simulink model "inner_pid_discrete_test"  (R2016a)
settings: Solver=VariableStepAuto  StartTime=0.0  StopTime=50  RelTol=1e-3
values from neighbouring files (symbols this model uses):
  max_ang_ref = 0.5    [init.m]
  PosD = 0.24    [init.m]
  PosI = 0    [init.m]
  PosP = 0.20    (= 0.2)    [init.m]
undefined symbols (not defined in the file or in its folder): b, inner_h, inner_maxlim, inner_minlim, k, l
libraries: simulink x7, vrlib x2

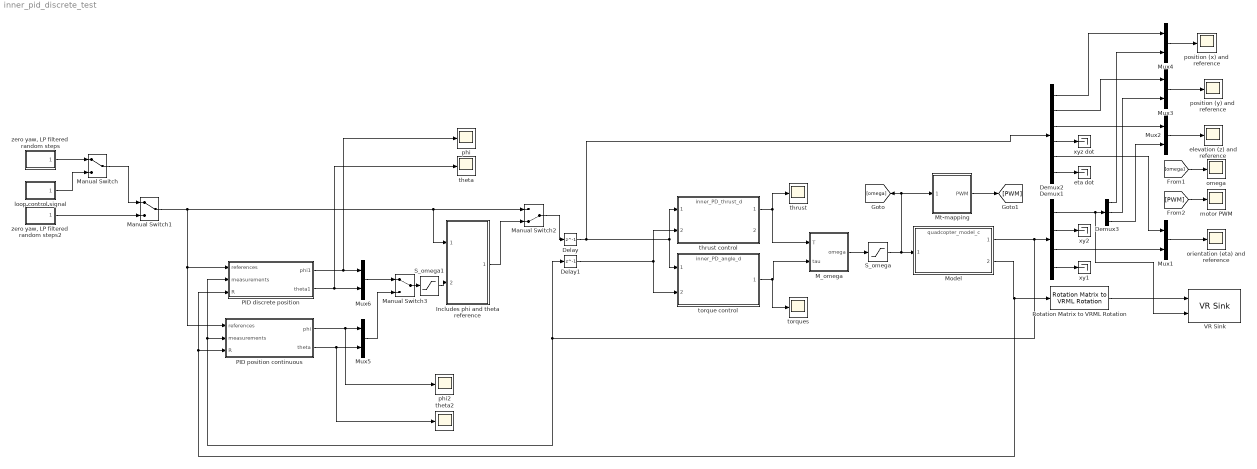
== system inner_pid_discrete_test ==
  "   eta dot" : Terminator
  "   xy1" : Terminator
  "   xy2" : Terminator
  "  xyz dot" : Terminator
  Delay : Delay  DelayLength=1  InitialCondition=0  SampleTime=inner_h
  Delay1 : Delay  DelayLength=1  InitialCondition=0  SampleTime=inner_h
  Demux1 : Demux  Outputs=[3,3,3,3]
  Demux2 : Demux  Outputs=[1,1,1,3,3,3]
  Demux3 : Demux  Outputs=[1,1,1]
  Includes phi and theta reference : Subsystem
  M_omega : Subsystem
  Manual Switch : ManualSwitch
  Manual Switch1 : ManualSwitch
  Manual Switch2 : ManualSwitch  CurrentSetting=0
  Manual Switch3 : ManualSwitch
  Model : ModelReference  ModelNameDialog=quadcopter_model_c.mdl  SimulationMode=Normal  ModelReferenceVersion=1.156
  Mt-mapping : Subsystem
  Mux{1..6} (6 alike) : Mux  Inputs=2
  PID discrete position : Subsystem
  PID position continuous : Subsystem
  Rotation Matrix to VRML Rotation : vrlib/Utilities/Rotation Matrix to VRML Rotation  maxzero=1e-12
  S_omega : Saturate  UpperLimit=inner_maxlim  LowerLimit=inner_minlim
  S_omega1 : Saturate
  VR Sink : vrlib/VR Sink  InstantiateOnLoad=on  SampleTime=0.1  ViewEnable=on  RemoteChange=off  RemoteView=off  FieldsWritten=copter.rotation.4.1.1.double#copter.translation.3.1.1.double  WorldFileName=copter_world.wrl  AutoView=on  VideoDimensions=[]  AllowVariableSize=off
  elevation (z) and reference : Scope
  loop control signal : Subsystem
  motor PWM : Scope
  "omega " : Scope
  orientation (eta) and reference : Scope
  phi : Scope
  phi2 : Scope
  position (x) and  reference : Scope
  position (y) and  reference : Scope
  theta : Scope
  theta2 : Scope
  thrust : Scope
  thrust control : ModelReference  ModelNameDialog=inner_PD_thrust_d.slx  SimulationMode=Normal  ModelReferenceVersion=1.81
  torque control : ModelReference  ModelNameDialog=inner_PD_angle_d.slx  SimulationMode=Normal  ModelReferenceVersion=1.85
  torques : Scope
  "zero yaw, LP filtered random steps" : Subsystem
  "zero yaw, LP filtered random steps2" : Subsystem
  wires:
  S_omega/1 -> [omega], Mt-mapping/1(omega), Model/1
  loop control signal/1(reference) -> Manual Switch/2
  "zero yaw, LP filtered random steps"/1(reference) -> Manual Switch/1
  Demux2/3 -> Mux2/1
  Mux2/1 -> elevation (z) and reference/1
  Mux1/1 -> orientation (eta) and reference/1
  Demux2/4 -> "  xyz dot"/1
  Demux2/6 -> "   eta dot"/1
  Demux2/1 -> Mux4/1
  Demux1/3 -> Mux1/2
  Demux1/1 -> VR Sink/2, Demux3/1
  [omega] -> "omega "/1
  Demux2/5 -> Mux1/1
  thrust control/1 -> thrust/1, M_omega/1(T)
  torque control/1 -> torques/1, M_omega/2(tau)
  M_omega/1(omega) -> S_omega/1
  Delay/1 -> Demux2/1, torque control/1, thrust control/1
  Delay1/1 -> thrust control/2, torque control/2
  Rotation Matrix to VRML Rotation/1 -> VR Sink/1
  Model/2 -> PID discrete position/3(R), PID position continuous/3(R), Rotation Matrix to VRML Rotation/1
  Demux1/4 -> "   xy1"/1
  Demux1/2 -> "   xy2"/1
  Demux3/3 -> Mux2/2
  Demux3/2 -> Mux3/2
  Mt-mapping/1(PWM) -> [PWM]
  [PWM] -> motor PWM/1
  Manual Switch/1 -> Manual Switch1/1
  "zero yaw, LP filtered random steps2"/1(reference) -> Manual Switch1/2
  Manual Switch1/1 -> Includes phi and theta reference/1(traj_reference), Manual Switch2/1, PID position continuous/1(references), PID discrete position/1(references)
  Manual Switch2/1 -> Delay/1
  Includes phi and theta reference/1(reference) -> Manual Switch2/2
  Mux3/1 -> position (y) and  reference/1
  Mux4/1 -> position (x) and  reference/1
  Demux3/1 -> Mux4/2
  Demux2/2 -> Mux3/1
  Model/1 -> Delay1/1, PID discrete position/2(measurements), PID position continuous/2(measurements), Demux1/1
  Mux5/1 -> Manual Switch3/2
  Mux6/1 -> Manual Switch3/1
  PID position continuous/1(phi) -> phi2/1, Mux5/1
  PID position continuous/2(theta) -> theta2/1, Mux5/2
  Manual Switch3/1 -> S_omega1/1
  S_omega1/1 -> Includes phi and theta reference/2(phi & theta)
  PID discrete position/1(phi1) -> phi/1, Mux6/1
  PID discrete position/2(theta1) -> theta/1, Mux6/2

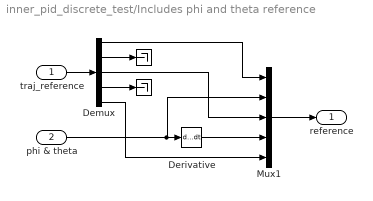
== system inner_pid_discrete_test/Includes phi and theta reference ==
  traj_reference : Inport
  phi & theta : Inport  Port=2
  " " : Terminator
  "  " : Terminator
  Demux : Demux  Outputs=[6,2,1,2,1]
  Derivative : Derivative
  Mux1 : Mux  Inputs=5
  reference : Outport
  wires:
  phi & theta/1 -> Mux1/2, Derivative/1
  traj_reference/1 -> Demux/1
  Demux/2 -> " "/1
  Demux/4 -> "  "/1
  Demux/1 -> Mux1/1
  Demux/3 -> Mux1/3
  Demux/5 -> Mux1/5
  Derivative/1 -> Mux1/4
  Mux1/1 -> reference/1

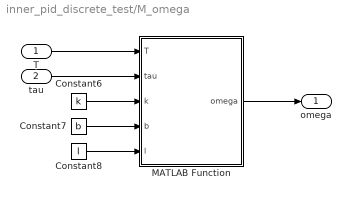
== system inner_pid_discrete_test/M_omega ==
  T : Inport
  tau : Inport  Port=2
  Constant6 : Constant  Value=k
  Constant7 : Constant  Value=b
  Constant8 : Constant  Value=l
  MATLAB Function : MATLAB Function  TreatAsAtomicUnit=on
  omega : Outport
  wires:
  Constant7/1 -> MATLAB Function/4(b)
  tau/1 -> MATLAB Function/2(tau)
  Constant6/1 -> MATLAB Function/3(k)
  MATLAB Function/1(omega) -> omega/1
  T/1 -> MATLAB Function/1(T)
  Constant8/1 -> MATLAB Function/5(l)

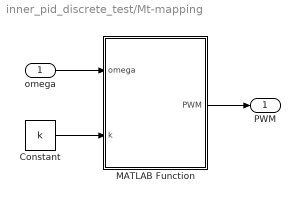
== system inner_pid_discrete_test/Mt-mapping ==
  omega : Inport
  Constant : Constant  Value=k
  MATLAB Function : MATLAB Function  TreatAsAtomicUnit=on
  PWM : Outport
  wires:
  MATLAB Function/1(PWM) -> PWM/1
  omega/1 -> MATLAB Function/1(omega)
  Constant/1 -> MATLAB Function/2(k)

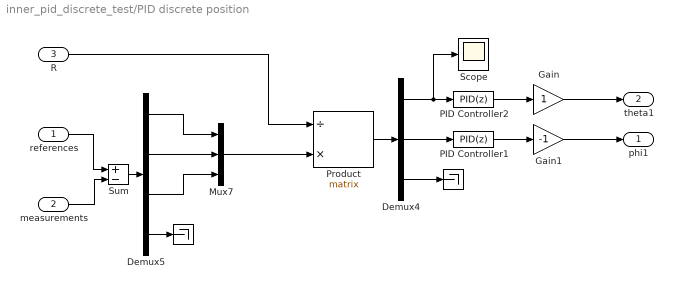
== system inner_pid_discrete_test/PID discrete position ==
  references : Inport
  measurements : Inport  Port=2
  R : Inport  Port=3
  "      " : Terminator
  "       " : Terminator
  Demux4 : Demux  Outputs=[1,1,1]
  Demux5 : Demux  Outputs=[1,1,1,9]
  Gain : Gain
  Gain1 : Gain  Gain=-1
  Mux7 : Mux  Inputs=3
  PID Controller1 : simulink/Continuous/PID Controller  Controller=PID  TimeDomain=Discrete-time  SampleTime=0.002  IntegratorMethod=Forward Euler  FilterMethod=Forward Euler  Form=Parallel  UseFilter=on  ControllerParametersSource=internal  P=PosP  I=PosI  D=PosD  N=100  InitialConditionSource=internal  InitialConditionForIntegrator=0  InitialConditionForFilter=0  ExternalReset=none  LimitOutput=off  UpperSaturationLimit=inf  LowerSaturationLimit=-inf  LinearizeAsGain=on  AntiWindupMode=none  Kb=1  TrackingMode=off  Kt=1  PParamMin=[]  PParamMax=[]  IParamMin=[]  IParamMax=[]  DParamMin=[]  DParamMax=[]  NParamMin=[]  NParamMax=[]  KbParamMin=[]  KbParamMax=[]  KtParamMin=[]  KtParamMax=[]  POutMin=[]  POutMax=[]  IOutMin=[]  IOutMax=[]  DOutMin=[]  DOutMax=[]  NOutMin=[]  NOutMax=[]  KbOutMin=[]  KbOutMax=[]  KtOutMin=[]  KtOutMax=[]  IntegratorOutMin=[]  IntegratorOutMax=[]  FilterOutMin=[]  FilterOutMax=[]  SumOutMin=[]  SumOutMax=[]  SumI1OutMin=[]  SumI1OutMax=[]  SumI2OutMin=[]  SumI2OutMax=[]  SumI3OutMin=[]  SumI3OutMax=[]  SumDOutMin=[]  SumDOutMax=[]  SaturationOutMin=[]  SaturationOutMax=[]  IntegratorContinuousStateAttributes=''  IntegratorStateMustResolveToSignalObject=off  IntegratorRTWStateStorageClass=Auto  FilterContinuousStateAttributes=''  FilterStateMustResolveToSignalObject=off  FilterRTWStateStorageClass=Auto  DifferentiatorICPrevScaledInput=0  DifferentiatorOutMin=[]  DifferentiatorOutMax=[]
  PID Controller2 : simulink/Continuous/PID Controller  Controller=PID  TimeDomain=Discrete-time  SampleTime=0.002  IntegratorMethod=Forward Euler  FilterMethod=Forward Euler  Form=Parallel  UseFilter=on  ControllerParametersSource=internal  P=PosP  I=PosI  D=PosD  N=100  InitialConditionSource=internal  InitialConditionForIntegrator=0  InitialConditionForFilter=0  ExternalReset=none  LimitOutput=off  UpperSaturationLimit=inf  LowerSaturationLimit=-inf  LinearizeAsGain=on  AntiWindupMode=none  Kb=1  TrackingMode=off  Kt=1  PParamMin=[]  PParamMax=[]  IParamMin=[]  IParamMax=[]  DParamMin=[]  DParamMax=[]  NParamMin=[]  NParamMax=[]  KbParamMin=[]  KbParamMax=[]  KtParamMin=[]  KtParamMax=[]  POutMin=[]  POutMax=[]  IOutMin=[]  IOutMax=[]  DOutMin=[]  DOutMax=[]  NOutMin=[]  NOutMax=[]  KbOutMin=[]  KbOutMax=[]  KtOutMin=[]  KtOutMax=[]  IntegratorOutMin=[]  IntegratorOutMax=[]  FilterOutMin=[]  FilterOutMax=[]  SumOutMin=[]  SumOutMax=[]  SumI1OutMin=[]  SumI1OutMax=[]  SumI2OutMin=[]  SumI2OutMax=[]  SumI3OutMin=[]  SumI3OutMax=[]  SumDOutMin=[]  SumDOutMax=[]  SaturationOutMin=[]  SaturationOutMax=[]  IntegratorContinuousStateAttributes=''  IntegratorStateMustResolveToSignalObject=off  IntegratorRTWStateStorageClass=Auto  FilterContinuousStateAttributes=''  FilterStateMustResolveToSignalObject=off  FilterRTWStateStorageClass=Auto  DifferentiatorICPrevScaledInput=0  DifferentiatorOutMin=[]  DifferentiatorOutMax=[]
  Product : Product  Inputs=/*  Multiplication=Matrix(*)
  Scope : Scope
  Sum : Sum  Inputs=+-
  phi1 : Outport
  theta1 : Outport  Port=2
  wires:
  Gain1/1 -> phi1/1
  Demux5/1 -> Mux7/1
  R/1 -> Product/1
  Gain/1 -> theta1/1
  Demux5/3 -> Mux7/3
  references/1 -> Sum/1
  Demux4/1 -> Scope/1, PID Controller2/1
  Sum/1 -> Demux5/1
  PID Controller2/1 -> Gain/1
  Demux4/2 -> PID Controller1/1
  Demux4/3 -> "       "/1
  measurements/1 -> Sum/2
  Demux5/4 -> "      "/1
  Demux5/2 -> Mux7/2
  Mux7/1 -> Product/2
  Product/1 -> Demux4/1
  PID Controller1/1 -> Gain1/1

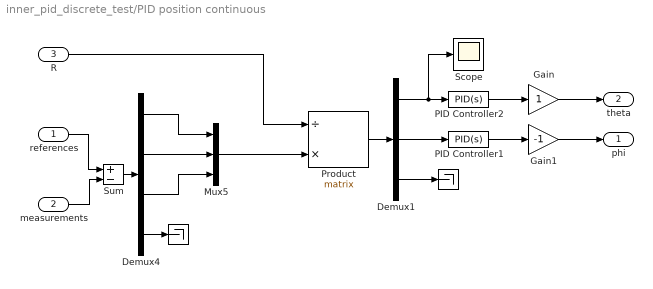
== system inner_pid_discrete_test/PID position continuous ==
  references : Inport
  measurements : Inport  Port=2
  R : Inport  Port=3
  "      " : Terminator
  "       " : Terminator
  Demux1 : Demux  Outputs=[1,1,1]
  Demux4 : Demux  Outputs=[1,1,1,9]
  Gain : Gain
  Gain1 : Gain  Gain=-1
  Mux5 : Mux  Inputs=3
  PID Controller1 : simulink/Continuous/PID Controller  Controller=PID  TimeDomain=Continuous-time  SampleTime=-1  IntegratorMethod=Forward Euler  FilterMethod=Forward Euler  Form=Parallel  UseFilter=on  ControllerParametersSource=internal  P=PosP  I=PosI  D=PosD  N=100  InitialConditionSource=internal  InitialConditionForIntegrator=0  InitialConditionForFilter=0  ExternalReset=none  LimitOutput=off  UpperSaturationLimit=inf  LowerSaturationLimit=-inf  LinearizeAsGain=on  AntiWindupMode=none  Kb=1  TrackingMode=off  Kt=1  PParamMin=[]  PParamMax=[]  IParamMin=[]  IParamMax=[]  DParamMin=[]  DParamMax=[]  NParamMin=[]  NParamMax=[]  KbParamMin=[]  KbParamMax=[]  KtParamMin=[]  KtParamMax=[]  POutMin=[]  POutMax=[]  IOutMin=[]  IOutMax=[]  DOutMin=[]  DOutMax=[]  NOutMin=[]  NOutMax=[]  KbOutMin=[]  KbOutMax=[]  KtOutMin=[]  KtOutMax=[]  IntegratorOutMin=[]  IntegratorOutMax=[]  FilterOutMin=[]  FilterOutMax=[]  SumOutMin=[]  SumOutMax=[]  SumI1OutMin=[]  SumI1OutMax=[]  SumI2OutMin=[]  SumI2OutMax=[]  SumI3OutMin=[]  SumI3OutMax=[]  SumDOutMin=[]  SumDOutMax=[]  SaturationOutMin=[]  SaturationOutMax=[]  IntegratorContinuousStateAttributes=''  IntegratorStateMustResolveToSignalObject=off  IntegratorRTWStateStorageClass=Auto  FilterContinuousStateAttributes=''  FilterStateMustResolveToSignalObject=off  FilterRTWStateStorageClass=Auto  DifferentiatorICPrevScaledInput=0  DifferentiatorOutMin=[]  DifferentiatorOutMax=[]
  PID Controller2 : simulink/Continuous/PID Controller  Controller=PID  TimeDomain=Continuous-time  SampleTime=-1  IntegratorMethod=Forward Euler  FilterMethod=Forward Euler  Form=Parallel  UseFilter=on  ControllerParametersSource=internal  P=PosP  I=PosI  D=PosD  N=100  InitialConditionSource=internal  InitialConditionForIntegrator=0  InitialConditionForFilter=0  ExternalReset=none  LimitOutput=off  UpperSaturationLimit=inf  LowerSaturationLimit=-inf  LinearizeAsGain=on  AntiWindupMode=none  Kb=1  TrackingMode=off  Kt=1  PParamMin=[]  PParamMax=[]  IParamMin=[]  IParamMax=[]  DParamMin=[]  DParamMax=[]  NParamMin=[]  NParamMax=[]  KbParamMin=[]  KbParamMax=[]  KtParamMin=[]  KtParamMax=[]  POutMin=[]  POutMax=[]  IOutMin=[]  IOutMax=[]  DOutMin=[]  DOutMax=[]  NOutMin=[]  NOutMax=[]  KbOutMin=[]  KbOutMax=[]  KtOutMin=[]  KtOutMax=[]  IntegratorOutMin=[]  IntegratorOutMax=[]  FilterOutMin=[]  FilterOutMax=[]  SumOutMin=[]  SumOutMax=[]  SumI1OutMin=[]  SumI1OutMax=[]  SumI2OutMin=[]  SumI2OutMax=[]  SumI3OutMin=[]  SumI3OutMax=[]  SumDOutMin=[]  SumDOutMax=[]  SaturationOutMin=[]  SaturationOutMax=[]  IntegratorContinuousStateAttributes=''  IntegratorStateMustResolveToSignalObject=off  IntegratorRTWStateStorageClass=Auto  FilterContinuousStateAttributes=''  FilterStateMustResolveToSignalObject=off  FilterRTWStateStorageClass=Auto  DifferentiatorICPrevScaledInput=0  DifferentiatorOutMin=[]  DifferentiatorOutMax=[]
  Product : Product  Inputs=/*  Multiplication=Matrix(*)
  Scope : Scope
  Sum : Sum  Inputs=+-
  phi : Outport
  theta : Outport  Port=2
  wires:
  PID Controller1/1 -> Gain1/1
  Sum/1 -> Demux4/1
  references/1 -> Sum/1
  measurements/1 -> Sum/2
  PID Controller2/1 -> Gain/1
  Gain/1 -> theta/1
  Demux4/3 -> Mux5/3
  Gain1/1 -> phi/1
  Demux4/4 -> "      "/1
  Demux4/2 -> Mux5/2
  Demux4/1 -> Mux5/1
  R/1 -> Product/1
  Mux5/1 -> Product/2
  Product/1 -> Demux1/1
  Demux1/2 -> PID Controller1/1
  Demux1/1 -> Scope/1, PID Controller2/1
  Demux1/3 -> "       "/1

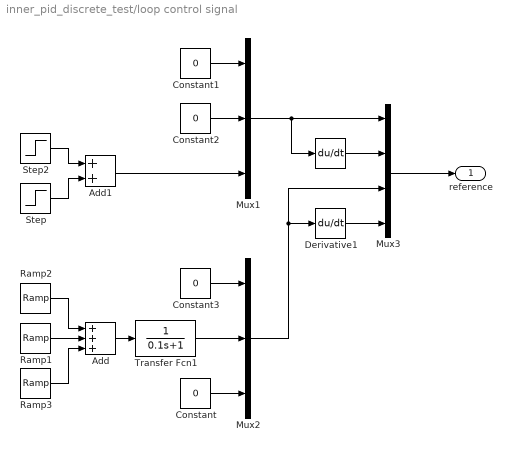
== system inner_pid_discrete_test/loop control signal ==
  "        " : Derivative
  Add : Sum  Inputs=+++
  Add1 : Sum
  Constant{,1..3} (4 alike) : Constant  Value=0
  Derivative1 : Derivative
  Mux1 : Mux  Inputs=3
  Mux2 : Mux  Inputs=3
  Mux3 : Mux  Inputs=[3,3,3,3]
  Ramp1 : simulink/Sources/Ramp  slope=2*2*pi  start=3.9  X0=0
  Ramp2 : simulink/Sources/Ramp  slope=-2*pi  start=5  X0=0
  Ramp3 : simulink/Sources/Ramp  slope=-2*pi  start=3.8  X0=0
  Step : Step  Time=5.5  After=-2  SampleTime=0
  Step2 : Step  Time=3.6  After=2  SampleTime=0
  Transfer Fcn1 : TransferFcn  Denominator=[0.1 1]
  reference : Outport
  wires:
  Mux1/1 -> "        "/1, Mux3/1
  Mux3/1 -> reference/1
  Derivative1/1 -> Mux3/4
  "        "/1 -> Mux3/2
  Mux2/1 -> Mux3/3, Derivative1/1
  Add/1 -> Transfer Fcn1/1
  Transfer Fcn1/1 -> Mux2/2
  Constant/1 -> Mux2/3
  Constant1/1 -> Mux1/1
  Constant2/1 -> Mux1/2
  Ramp2/1 -> Add/1
  Ramp1/1 -> Add/2
  Step2/1 -> Add1/1
  Step/1 -> Add1/2
  Ramp3/1 -> Add/3
  Constant3/1 -> Mux2/1
  Add1/1 -> Mux1/3

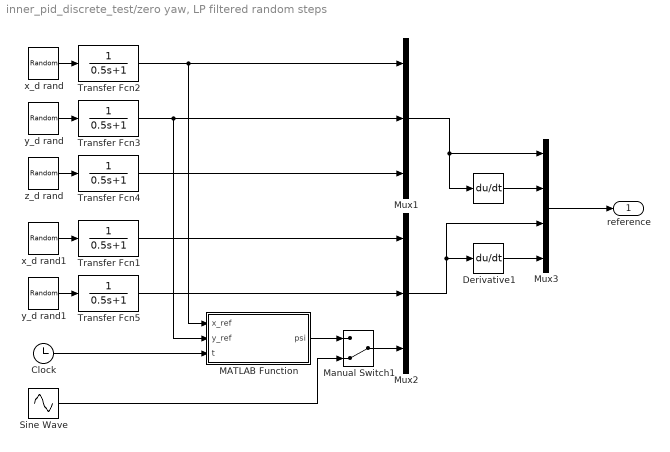
== system inner_pid_discrete_test/zero yaw, LP filtered random steps ==
  "        " : Derivative
  Clock : Clock
  Derivative1 : Derivative
  MATLAB Function : MATLAB Function  TreatAsAtomicUnit=on
  Manual Switch1 : ManualSwitch  CurrentSetting=0
  Mux1 : Mux  Inputs=3
  Mux2 : Mux  Inputs=3
  Mux3 : Mux  Inputs=[3,3,3,3]
  Sine Wave : Sin  Amplitude=0.5  Frequency=0.5  SampleTime=0
  Transfer Fcn{1..5} (5 alike) : TransferFcn  Denominator=[0.5 1]
  x_d rand : UniformRandomNumber  Minimum=-3  Maximum=3  Seed=6  SampleTime=10
  x_d rand1 : UniformRandomNumber  Minimum=-0.1  Maximum=0.1  SampleTime=10
  y_d rand : UniformRandomNumber  Minimum=-3  Maximum=3  Seed=4  SampleTime=10
  y_d rand1 : UniformRandomNumber  Minimum=-0.1  Maximum=0.1  Seed=1  SampleTime=10
  z_d rand : UniformRandomNumber  Minimum=0  Maximum=3  Seed=2  SampleTime=10
  reference : Outport
  wires:
  Mux1/1 -> "        "/1, Mux3/1
  Mux3/1 -> reference/1
  Derivative1/1 -> Mux3/4
  "        "/1 -> Mux3/2
  Mux2/1 -> Mux3/3, Derivative1/1
  Transfer Fcn1/1 -> Mux2/1
  Transfer Fcn5/1 -> Mux2/2
  Manual Switch1/1 -> Mux2/3
  x_d rand/1 -> Transfer Fcn2/1
  y_d rand/1 -> Transfer Fcn3/1
  z_d rand/1 -> Transfer Fcn4/1
  Transfer Fcn2/1 -> Mux1/1, MATLAB Function/1(x_ref)
  Transfer Fcn3/1 -> Mux1/2, MATLAB Function/2(y_ref)
  Transfer Fcn4/1 -> Mux1/3
  x_d rand1/1 -> Transfer Fcn1/1
  y_d rand1/1 -> Transfer Fcn5/1
  MATLAB Function/1(psi) -> Manual Switch1/1
  Sine Wave/1 -> Manual Switch1/2
  Clock/1 -> MATLAB Function/3(t)

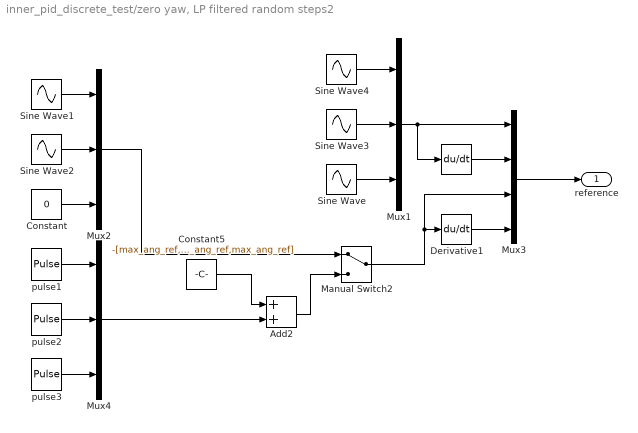
== system inner_pid_discrete_test/zero yaw, LP filtered random steps2 ==
  "        " : Derivative
  Add2 : Sum
  Constant : Constant  Value=0
  Constant5 : Constant  Value=-[max_ang_ref,max_ang_ref,max_ang_ref]
  Derivative1 : Derivative
  Manual Switch2 : ManualSwitch
  Mux1 : Mux  Inputs=3
  Mux2 : Mux  Inputs=3
  Mux3 : Mux  Inputs=[3,3,3,3]
  Mux4 : Mux  Inputs=3
  Sine Wave : Sin  Bias=2  SampleTime=0
  Sine Wave1 : Sin  Amplitude=max_ang_ref  SampleTime=0
  Sine Wave2 : Sin  Amplitude=max_ang_ref  Phase=pi/2
  Sine Wave3 : Sin  Phase=pi/2  SampleTime=0
  Sine Wave4 : Sin  Frequency=0.6  SampleTime=0
  pulse1 : DiscretePulseGenerator  PulseType=Time based  Amplitude=max_ang_ref*2  Period=10  PulseWidth=50
  pulse2 : DiscretePulseGenerator  PulseType=Time based  Amplitude=max_ang_ref*2  Period=10  PulseWidth=50
  pulse3 : DiscretePulseGenerator  PulseType=Time based  Amplitude=max_ang_ref*2  Period=10  PulseWidth=50
  reference : Outport
  wires:
  Mux1/1 -> "        "/1, Mux3/1
  Mux3/1 -> reference/1
  Derivative1/1 -> Mux3/4
  "        "/1 -> Mux3/2
  Sine Wave1/1 -> Mux2/1
  Sine Wave2/1 -> Mux2/2
  Constant/1 -> Mux2/3
  Sine Wave/1 -> Mux1/3
  pulse1/1 -> Mux4/1
  pulse2/1 -> Mux4/2
  pulse3/1 -> Mux4/3
  Constant5/1 -> Add2/1
  Mux4/1 -> Add2/2
  Mux2/1 -> Manual Switch2/1
  Add2/1 -> Manual Switch2/2
  Manual Switch2/1 -> Mux3/3, Derivative1/1
  Sine Wave3/1 -> Mux1/2
  Sine Wave4/1 -> Mux1/1

== matlab function inner_pid_discrete_test/zero yaw, LP filtered random steps/MATLAB Function ==
function psi = scan(x_ref, y_ref, t)
%#codegen
psi = atan2(x_ref, y_ref) + 0.3*sin(0.5*t);

== matlab function inner_pid_discrete_test/M_omega/MATLAB Function ==
function omega = Mw(T, tau, k, b, l)
%#codegen
tau_phi = tau(1);
tau_theta = tau(2);
tau_psi = tau(3);
w1sq = T/(4*k) - tau_theta/(2*k*l) - tau_psi / (4*b);
w2sq = T/(4*k) - tau_phi/(2*k*l) + tau_psi / (4*b);
w3sq = T/(4*k) + tau_theta/(2*k*l) - tau_psi / (4*b);
w4sq = T/(4*k) + tau_phi/(2*k*l) + tau_psi / (4*b);

omega = sqrt(max([w1sq w2sq w3sq w4sq]', 0));

== matlab function inner_pid_discrete_test/Mt-mapping/MATLAB Function ==
function PWM = Mt(omega, k)
%#codegen
rotor_thrusts = k.*omega.^2;
beta1 = 0.0877;
beta2 = 0.0660;
PWM =  -beta1/(2*beta2) + sqrt((beta1/(2*beta2))^2 + rotor_thrusts/beta2);
